simulink model "Quadrotor_14_step0_code_gen"  (Simulink 7.6)
settings: Solver=ode8  StartTime=0.0  StopTime=500  RelTol=1e-3
undefined symbols (not defined in the file): STARMAC, uav_utilities
libraries: aero_sim_lib x8, passive_control x1, simulink x1
settings Model: Creator=fluffy_bear  LastModifiedBy=jporter
settings OptimizationCC: BlockReduction=off  EnhancedBackFolding=on  OptimizeModelRefInitCode=on  LifeSpan=1
settings HardwareCC: ProdLargestAtomicInteger=Long  ProdLargestAtomicFloat=Float  ProdIntDivRoundTo=Floor  ProdEndianess=LittleEndian  ProdHWDeviceType=ARM Compatible->ARM 7
settings SFSimCC: SimParseCustomCode=off
settings RTWCC: SystemTargetFile=ert.tlc  GenCodeOnly=on  TemplateMakefile=ert_default_tmf  Description=Real-Time Workshop Embedded Coder  GenerateReport=on  ProcessScript=ert_make_rtw_hook  IncludeHyperlinkInReport=on  LaunchReport=on  CheckMdlBeforeBuild=Warning
settings CodeAppCC: IgnoreCustomStorageClasses=off  MATLABSourceComments=on
settings ERTTargetCC: MultiwordLength=2048  GenerateSampleERTMain=on  CombineSignalStateStructs=on  MultiInstanceERTCode=on  MultiInstanceErrorCode=Warning  ERTCustomFileTemplate=example_file_process.tlc  ConvertIfToSwitch=off

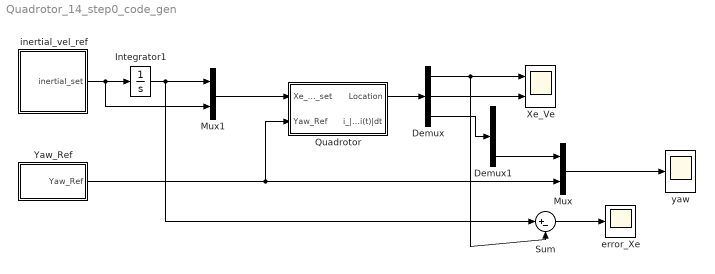
== system Quadrotor_14_step0_code_gen ==
  Demux : Demux  Outputs=[3,3,3]
  Demux1 : Demux  Outputs=3
  Integrator1 : Integrator
  Mux : Mux  Inputs=2
  Mux1 : Mux  Inputs=2
  Quadrotor : Subsystem  AncestorBlock=uav_utilities/STARMAC
  Sum : Sum  Inputs=|+-
  Xe_Ve : Scope  NumInputPorts=2
      settings: YMin=-100~-1.75  YMax=100~1.75  MaxDataPoints=100000  SampleInput=on  SampleTime=100/5000
  Yaw_Ref : Subsystem
  error_Xe : Scope
      settings: YMin=-9  SaveName=error_data  MaxDataPoints=20000  Decimation=10  SampleInput=on  SampleTime=100/5000
  inertial_vel_ref : Subsystem
  yaw : Scope
      settings: TimeRange=2  YMin=0.325  YMax=0.9  MaxDataPoints=100000  SampleInput=on  SampleTime=100/5000
  wires:
  inertial_vel_ref/1(inertial_set) -> Integrator1/1, Mux1/2
  Yaw_Ref/1(Yaw_Ref) -> Quadrotor/2(Yaw_Ref), Mux/2
  Sum/1 -> error_Xe/1
  Quadrotor/1(Location) -> Demux/1
  Demux/1 -> Sum/2, Xe_Ve/1
  Demux/2 -> Xe_Ve/2
  Mux/1 -> yaw/1
  Demux/3 -> Demux1/1
  Demux1/3 -> Mux/1
  Integrator1/1 -> Mux1/1, Sum/1
  Mux1/1 -> Quadrotor/1(Xe_Ve_set)

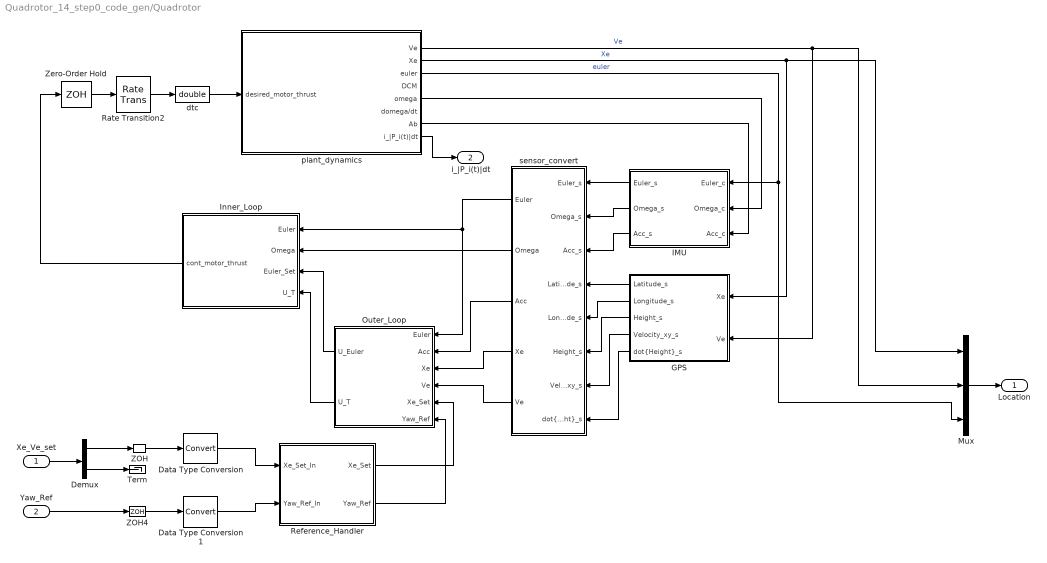
== system Quadrotor_14_step0_code_gen/Quadrotor ==
  Xe_Ve_set : Inport  PortDimensions=[6]
  Yaw_Ref : Inport  Port=2  PortDimensions=[1]
  Data Type Conversion : DataTypeConversion
  Data Type Conversion1 : DataTypeConversion
  Demux : Demux  Outputs=[3,3]
  GPS : Subsystem
  IMU : Subsystem
  Inner_Loop : Subsystem
  Mux : Mux  Inputs=[3 3 3]
  Outer_Loop : Subsystem
  Rate Transition2 : RateTransition
  Reference_Handler : Subsystem
  Term : Terminator
  ZOH : ZeroOrderHold  SampleTime=.01
  ZOH4 : ZeroOrderHold  SampleTime=.01
  Zero-Order Hold : ZeroOrderHold  SampleTime=.02
  dtc : DataTypeConversion  OutDataTypeStr=double
  plant_dynamics : Subsystem  AncestorBlock=aero_sim_lib/starmac_dynamics
  sensor_convert : Subsystem
  Location : Outport
  i_|P_i(t)|dt : Outport  Port=2
  wires:
  ZOH4/1 -> Data Type Conversion1/1
  Demux/2 -> Term/1
  Demux/1 -> ZOH/1
  Xe_Ve_set/1 -> Demux/1
  Mux/1 -> Location/1
  plant_dynamics/3(euler) -> Mux/3, IMU/1(Euler_c)  "euler"
  plant_dynamics/2(Xe) -> Mux/1, GPS/1(Xe)  "Xe"
  plant_dynamics/1(Ve) -> Mux/2, GPS/2(Ve)  "Ve"
  dtc/1 -> plant_dynamics/1(desired_motor_thrust)
  Zero-Order Hold/1 -> Rate Transition2/1
  Rate Transition2/1 -> dtc/1
  ZOH/1 -> Data Type Conversion/1
  plant_dynamics/5(omega) -> IMU/2(Omega_c)
  plant_dynamics/7(Ab) -> IMU/3(Acc_c)
  plant_dynamics/8(i_|P_i(t)|dt) -> i_|P_i(t)|dt/1
  Yaw_Ref/1 -> ZOH4/1
  IMU/1(Euler_s) -> sensor_convert/1(Euler_s)
  IMU/2(Omega_s) -> sensor_convert/2(Omega_s)
  IMU/3(Acc_s) -> sensor_convert/3(Acc_s)
  GPS/1(Latitude_s) -> sensor_convert/4(Latitude_s)
  GPS/2(Longitude_s) -> sensor_convert/5(Longitude_s)
  GPS/3(Height_s) -> sensor_convert/6(Height_s)
  GPS/4(Velocity_xy_s) -> sensor_convert/7(Velocity_xy_s)
  GPS/5("dot{Height}_s") -> sensor_convert/8("dot{Height}_s")
  Outer_Loop/1(U_Euler) -> Inner_Loop/3(Euler_Set)
  Outer_Loop/2(U_T) -> Inner_Loop/4(U_T)
  sensor_convert/1(Euler) -> Inner_Loop/1(Euler), Outer_Loop/1(Euler)
  sensor_convert/2(Omega) -> Inner_Loop/2(Omega)
  sensor_convert/3(Acc) -> Outer_Loop/2(Acc)
  sensor_convert/4(Xe) -> Outer_Loop/3(Xe)
  sensor_convert/5(Ve) -> Outer_Loop/4(Ve)
  Data Type Conversion/1 -> Reference_Handler/1(Xe_Set_In)
  Data Type Conversion1/1 -> Reference_Handler/2(Yaw_Ref_In)
  Reference_Handler/1(Xe_Set) -> Outer_Loop/5(Xe_Set)
  Reference_Handler/2(Yaw_Ref) -> Outer_Loop/6(Yaw_Ref)
  Inner_Loop/1(cont_motor_thrust) -> Zero-Order Hold/1

== system Quadrotor_14_step0_code_gen/Yaw_Ref ==
  Signal Generator : SignalGenerator  Frequency=2*.0625*0.25
  Yaw_Ref : Outport
  wires:
  Signal Generator/1 -> Yaw_Ref/1

== system Quadrotor_14_step0_code_gen/inertial_vel_ref ==
  Signal Generator : SignalGenerator  Amplitude=1.8*[1 -1 -.5]  Frequency=.1*.0625*ones(3,1)
  inertial_set : Outport
  wires:
  Signal Generator/1 -> inertial_set/1

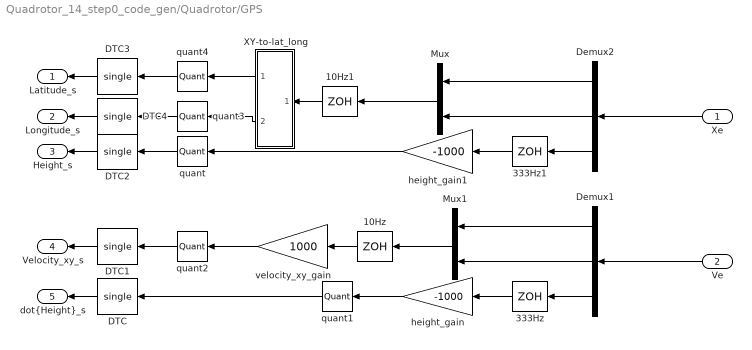
== system Quadrotor_14_step0_code_gen/Quadrotor/GPS ==
  Xe : Inport  OutDataTypeStr=double
  Ve : Inport  Port=2  OutDataTypeStr=double
  10Hz : ZeroOrderHold  SampleTime=.1
  10Hz1 : ZeroOrderHold  SampleTime=.1
  333Hz : ZeroOrderHold  SampleTime=1/333
  333Hz1 : ZeroOrderHold  SampleTime=1/333
  DTC{,1..4} (5 alike) : DataTypeConversion  OutDataTypeStr=single
  Demux1 : Demux  Outputs=[1,1,1]
  Demux2 : Demux  Outputs=[1,1,1]
  Mux : Mux  Inputs=2
  Mux1 : Mux  Inputs=2
  XY-to-lat_long : Subsystem  mask{lat_0=36.1658333, lon_0=-86.7844444}
  height_gain : Gain  Gain=-1000  RndMeth=Round  SaturateOnIntegerOverflow=on  OutDataTypeStr=Inherit: Same as input  LockScale=on
  height_gain1 : Gain  Gain=-1000  RndMeth=Round  SaturateOnIntegerOverflow=on  OutDataTypeStr=Inherit: Same as input  LockScale=on
  quant{,1,3..4} (4 alike) : Quantizer  QuantizationInterval=1
  quant2 : Quantizer  QuantizationInterval=ones(2,1)
  velocity_xy_gain : Gain  Gain=1000  RndMeth=Round  SaturateOnIntegerOverflow=on  OutDataTypeStr=Inherit: Same as input  LockScale=on
  Latitude_s : Outport
  Longitude_s : Outport  Port=2
  Height_s : Outport  Port=3
  Velocity_xy_s : Outport  Port=4
  "dot{Height}_s" : Outport  Port=5
  wires:
  Ve/1 -> Demux1/1
  Xe/1 -> Demux2/1
  Demux1/3 -> 333Hz/1
  Demux2/3 -> 333Hz1/1
  Demux2/1 -> Mux/1
  Demux2/2 -> Mux/2
  Demux1/1 -> Mux1/1
  Demux1/2 -> Mux1/2
  333Hz1/1 -> height_gain1/1
  333Hz/1 -> height_gain/1
  Mux1/1 -> 10Hz/1
  10Hz/1 -> velocity_xy_gain/1
  height_gain1/1 -> quant/1
  height_gain/1 -> quant1/1
  quant/1 -> DTC2/1
  quant1/1 -> DTC/1
  velocity_xy_gain/1 -> quant2/1
  quant2/1 -> DTC1/1
  10Hz1/1 -> XY-to-lat_long/1(XY)
  XY-to-lat_long/1(lat) -> quant4/1
  XY-to-lat_long/2(lon) -> quant3/1
  Mux/1 -> 10Hz1/1
  DTC/1 -> "dot{Height}_s"/1
  DTC1/1 -> Velocity_xy_s/1
  DTC2/1 -> Height_s/1
  DTC3/1 -> Latitude_s/1
  DTC4/1 -> Longitude_s/1
  quant3/1 -> DTC4/1
  quant4/1 -> DTC3/1

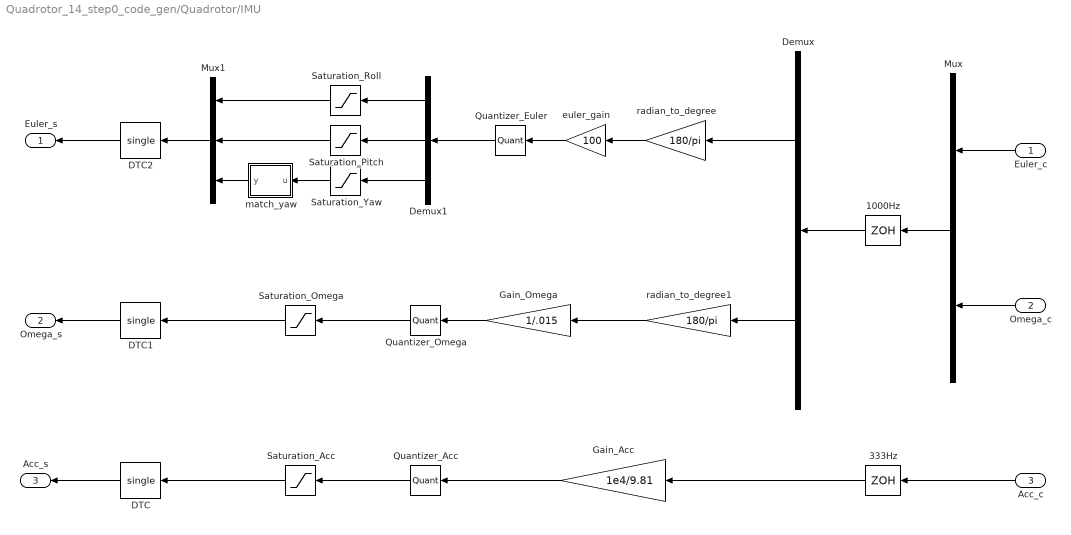
== system Quadrotor_14_step0_code_gen/Quadrotor/IMU ==
  Euler_c : Inport  OutDataTypeStr=double
  Omega_c : Inport  Port=2  OutDataTypeStr=double
  Acc_c : Inport  Port=3
  1000Hz : ZeroOrderHold  SampleTime=.001
  333Hz : ZeroOrderHold  SampleTime=1/333
  DTC : DataTypeConversion  OutDataTypeStr=single
  DTC1 : DataTypeConversion  OutDataTypeStr=single
  DTC2 : DataTypeConversion  OutDataTypeStr=single
  Demux : Demux  Outputs=[3,3]
  Demux1 : Demux  Outputs=[1,1,1]
  Gain_Acc : Gain  Gain=1e4/9.81
  Gain_Omega : Gain  Gain=1/.015
  Mux : Mux  Inputs=[3,3]
  Mux1 : Mux  Inputs=[1,1,1]
  Quantizer_Acc : Quantizer  QuantizationInterval=ones(3,1)
  Quantizer_Euler : Quantizer  QuantizationInterval=ones(3,1)
  Quantizer_Omega : Quantizer  QuantizationInterval=ones(3,1)
  Saturation_Acc : Saturate  UpperLimit=30000  LowerLimit=-30000  RndMeth=Round
      settings: LockScale=on
  Saturation_Omega : Saturate  UpperLimit=((2^15)-1) * ones(3,1)  LowerLimit=-(2^15) * ones(3,1)  OutDataTypeStr=double  RndMeth=Round
      settings: LockScale=on
  Saturation_Pitch : Saturate  UpperLimit=90*100  LowerLimit=-90*100  RndMeth=Round
      settings: LockScale=on
  Saturation_Roll : Saturate  UpperLimit=90*100  LowerLimit=-90*100  RndMeth=Round
      settings: LockScale=on
  Saturation_Yaw : Saturate  UpperLimit=180*100  LowerLimit=-180*100  RndMeth=Round
      settings: LockScale=on
  euler_gain : Gain  Gain=100
  match_yaw : Stateflow chart  TreatAsAtomicUnit=on
  radian_to_degree : Gain  Gain=180/pi
  radian_to_degree1 : Gain  Gain=180/pi
  Euler_s : Outport  LockScale=on
  Omega_s : Outport  Port=2  LockScale=on
  Acc_s : Outport  Port=3  LockScale=on
  wires:
  Mux/1 -> 1000Hz/1
  Euler_c/1 -> Mux/1
  1000Hz/1 -> Demux/1
  Gain_Acc/1 -> Quantizer_Acc/1
  Omega_c/1 -> Mux/2
  333Hz/1 -> Gain_Acc/1
  Saturation_Acc/1 -> DTC/1
  Saturation_Omega/1 -> DTC1/1
  Demux1/1 -> Saturation_Roll/1
  Saturation_Roll/1 -> Mux1/1
  Mux1/1 -> DTC2/1
  Demux1/2 -> Saturation_Pitch/1
  Saturation_Pitch/1 -> Mux1/2
  Demux1/3 -> Saturation_Yaw/1
  Saturation_Yaw/1 -> match_yaw/1(u)
  Gain_Omega/1 -> Quantizer_Omega/1
  Demux/1 -> radian_to_degree/1
  radian_to_degree/1 -> euler_gain/1
  Demux/2 -> radian_to_degree1/1
  euler_gain/1 -> Quantizer_Euler/1
  Quantizer_Euler/1 -> Demux1/1
  match_yaw/1(y) -> Mux1/3
  radian_to_degree1/1 -> Gain_Omega/1
  Quantizer_Omega/1 -> Saturation_Omega/1
  Acc_c/1 -> 333Hz/1
  Quantizer_Acc/1 -> Saturation_Acc/1
  DTC/1 -> Acc_s/1
  DTC1/1 -> Omega_s/1
  DTC2/1 -> Euler_s/1

== system Quadrotor_14_step0_code_gen/Quadrotor/Inner_Loop ==
  Euler : Inport  OutDataTypeStr=single
  Omega : Inport  Port=2  OutDataTypeStr=single
  Euler_Set : Inport  Port=3  OutDataTypeStr=single
  U_T : Inport  Port=4  OutDataTypeStr=single
  euler_controller : Subsystem  mask{K=1, K_e=7.5/.65, K_o=.5}
      mask prompts: K "Loop Gain [K]:"; K_e "Euler Gain [K_e]:"; K_o "Omega Gain [K_o]:"
  lead_motor : Subsystem  mask{tau_motor=.10, t_s=.01}
      mask init:
      | Hs=tf([tau_motor 1],[t_s/pi 1]);
      | Hz=ipesh_transform(Hs,t_s);
      | %a=1/tau_motor;
      | %b=pi/t_s;
      | %T=t_s;
      | %num1=b*(1-exp(-b*T))+a*(b*T-1+exp(-b*T));
      | %num2=-b*(1-exp(-b*T))+a*(1-exp(-b*T)-b*T*exp(-b*T));
      | %den1=a*b;
      | %den2=-a*b*exp(-b*T);
      | %num=[num1 num2];
      | %den=[den1 den2];
      | %Hz=tf(num,den,T);
      | %[y,t]=step(Hz);
      | %k_ss=(1/y(length(y)));
      | %num=k_ss*num;
      | %lead_a_1=single(-den(2)/den(1))
      | %lead_b_1=single(num(2)/den(1))
      | %lead_b_2=single(num(1)/den(1))
      | %Hz=k_ss*Hz
      | %bode(Hz);
  thrust_limit : Saturate  UpperLimit=10*ones(4,1)  LowerLimit=0*ones(4,1)  OutDataTypeStr=single
  u_T_u_torque_motor_thrust : Subsystem  mask{dx=.3048, K_torque=.47}
      mask prompts: dx "X distance of motor from CG [dx](meters):"; K_torque "Ktorque [K_torque]:"
      mask init:
      | M=[0 -dx 0 dx;
      |    dx 0 -dx 0;
      |    -K_torque K_torque -K_torque K_torque;
      |    1 1 1 1];
      | Mi=single(inv(M));
  cont_motor_thrust : Outport
  wires:
  Euler_Set/1 -> euler_controller/1(euler_set)
  U_T/1 -> u_T_u_torque_motor_thrust/2(u_T)
  euler_controller/1(u_torque) -> u_T_u_torque_motor_thrust/1(u_torque)
  thrust_limit/1 -> cont_motor_thrust/1
  u_T_u_torque_motor_thrust/1(cont_motor_thrust) -> lead_motor/1(thrust_in)
  lead_motor/1(thrust_out) -> thrust_limit/1
  Euler/1 -> euler_controller/2(euler)
  Omega/1 -> euler_controller/3(omega)

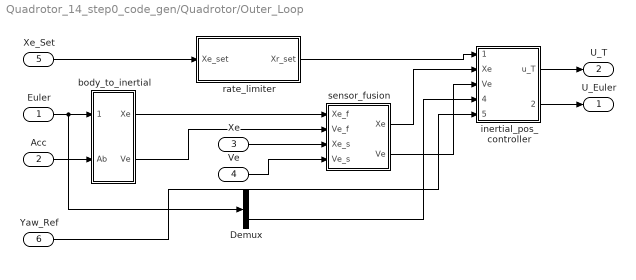
== system Quadrotor_14_step0_code_gen/Quadrotor/Outer_Loop ==
  Euler : Inport  OutDataTypeStr=single  PortDimensions=[3]
  Acc : Inport  Port=2  OutDataTypeStr=single  PortDimensions=[3]
  Xe : Inport  Port=3  OutDataTypeStr=single  PortDimensions=[3]
  Ve : Inport  Port=4  OutDataTypeStr=single  PortDimensions=[3]
  Xe_Set : Inport  Port=5  OutDataTypeStr=single  PortDimensions=[3]
  Yaw_Ref : Inport  Port=6  OutDataTypeStr=single  PortDimensions=[1]
  Demux : Demux  Outputs=3
  body_to_inertial : Subsystem
  inertial_pos_controller : Subsystem
  rate_limiter : Subsystem  mask{wn=2*pi, zeta=0.9, Vmax=2, T=0.01}
      mask prompts: wn "omega_n"; Vmax "Max velocity"; T "Sample time"
      mask init:
      | Hs=tf([wn^2],[1,2*zeta*wn,wn^2]);
      | Hz=ipesh_transform(Hs,T);
  sensor_fusion : Subsystem  mask{tau=.1, Ts=.01, Ts_gps=.1}
      mask prompts: tau "low-pass time constant (sec) [tau]"; Ts "Sample time [Ts]"; Ts_gps "GPS Sample Time [Ts_gps]"
  U_Euler : Outport  OutDataTypeStr=single  PortDimensions=[3]
  U_T : Outport  Port=2  OutDataTypeStr=single  PortDimensions=[1]
  wires:
  Xe_Set/1 -> rate_limiter/1(Xe_set)
  inertial_pos_controller/1(u_T) -> U_T/1
  inertial_pos_controller/2(u_euler) -> U_Euler/1
  Euler/1 -> body_to_inertial/1(euler), Demux/1
  Acc/1 -> body_to_inertial/2(Ab)
  sensor_fusion/1(Xe) -> inertial_pos_controller/2(Xe)
  sensor_fusion/2(Ve) -> inertial_pos_controller/3(Ve)
  body_to_inertial/1(Xe) -> sensor_fusion/1(Xe_f)
  body_to_inertial/2(Ve) -> sensor_fusion/2(Ve_f)
  Xe/1 -> sensor_fusion/3(Xe_s)
  Ve/1 -> sensor_fusion/4(Ve_s)
  rate_limiter/1(Xr_set) -> inertial_pos_controller/1(Xe_set)
  Demux/3 -> inertial_pos_controller/4(Yaw_actual)
  Yaw_Ref/1 -> inertial_pos_controller/5(Yaw_set)

== system Quadrotor_14_step0_code_gen/Quadrotor/Reference_Handler ==
  Xe_Set_In : Inport
  Yaw_Ref_In : Inport  Port=2
  Gain : Gain
  Gain1 : Gain
  Xe_Set : Outport
  Yaw_Ref : Outport  Port=2
  wires:
  Xe_Set_In/1 -> Gain/1
  Yaw_Ref_In/1 -> Gain1/1
  Gain1/1 -> Yaw_Ref/1
  Gain/1 -> Xe_Set/1

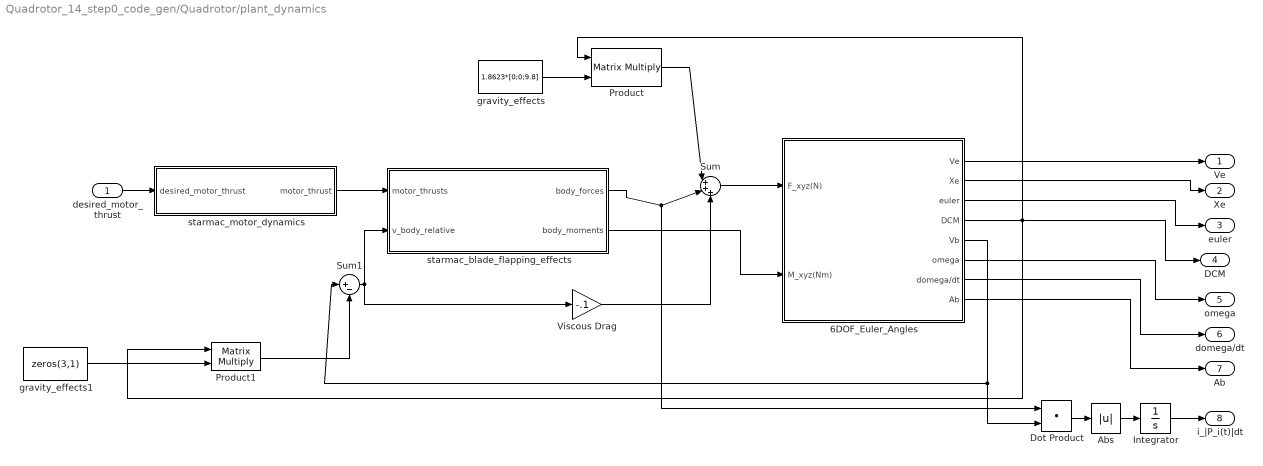
== system Quadrotor_14_step0_code_gen/Quadrotor/plant_dynamics ==
  desired_motor_thrust : Inport
  6DOF_Euler_Angles : Subsystem  AncestorBlock=aero_sim_lib/6DOF (Euler Angles)_CMU  mask{XYZe_0=[0.01;0.01;0], Vb_0=[0;0;0], euler_0=[0;0;0], omega_0=[0;0;0], M=1.8623, I=diag([0.02759 0.02771 0.04806])}
      mask prompts: XYZe_0 "Initial position in inertial axes [Xe,Ye,Ze]:"; Vb_0 "Initial velocity in body axes [U,v,w]:"; euler_0 "Initial Euler orientation [roll, pitch, yaw]=[phi,theta,psi]:"; omega_0 "Initial body rotation rates [p,q,r]=omega:"; M "Initial mass:"; I "Inertial:"
  Abs : Abs
  Dot Product : DotProduct  InputSameDT=on  OutDataTypeStr=Inherit: Inherit via internal rule
  Integrator : Integrator
  Product : Product  Multiplication=Matrix(*)  RndMeth=Zero
  Product1 : Product  Multiplication=Matrix(*)  RndMeth=Zero
  Sum : Sum  Inputs=|+++
  Sum1 : Sum  Inputs=|+-
  Viscous Drag : Gain  Gain=-.1
  gravity_effects : Constant  Value=1.8623*[0;0;9.8]
  gravity_effects1 : Constant  Value=zeros(3,1)  OutDataTypeStr=double
  starmac_blade_flapping_effects : Subsystem  AncestorBlock=aero_sim_lib/starmac_blade_flapping_effects
  starmac_motor_dynamics : Subsystem  AncestorBlock=aero_sim_lib/starmac_motor_dynamics  mask{tau_motor=.1, T_nom=1.8263*9.8/4, thrust_max=9.8, thrust_min=0, motor_lag_enable=on, motor_variance=.01*(.05*9.8/4)^2, Ts=1/76}
      mask prompts: tau_motor "tau_motor (seconds):"; T_nom "nominal thrust (N):"; thrust_max "maximum thrust (N):"; thrust_min "minimum thrust (N):"; motor_lag_enable "Motor Lag Enabled:"; motor_variance "Motor Variance [motor_variance]:"; Ts "Motor Update Rate (seconds):"
  Ve : Outport
  Xe : Outport  Port=2
  euler : Outport  Port=3
  DCM : Outport  Port=4
  omega : Outport  Port=5
  domega/dt : Outport  Port=6
  Ab : Outport  Port=7
  i_|P_i(t)|dt : Outport  Port=8
  wires:
  desired_motor_thrust/1 -> starmac_motor_dynamics/1(desired_motor_thrust)
  starmac_blade_flapping_effects/1(body_forces) -> Sum/2, Dot Product/1
  starmac_blade_flapping_effects/2(body_moments) -> 6DOF_Euler_Angles/2(M_xyz(Nm))
  Viscous Drag/1 -> Sum/3
  6DOF_Euler_Angles/5(Vb) -> Sum1/1, Dot Product/2
  Product1/1 -> Sum1/2
  Sum1/1 -> Viscous Drag/1, starmac_blade_flapping_effects/2(v_body_relative)
  gravity_effects/1 -> Product/2
  6DOF_Euler_Angles/4(DCM) -> Product1/1, Product/1, DCM/1
  Sum/1 -> 6DOF_Euler_Angles/1(F_xyz(N))
  Product/1 -> Sum/1
  starmac_motor_dynamics/1(motor_thrust) -> starmac_blade_flapping_effects/1(motor_thrusts)
  6DOF_Euler_Angles/1(Ve) -> Ve/1
  6DOF_Euler_Angles/2(Xe) -> Xe/1
  6DOF_Euler_Angles/3(euler) -> euler/1
  6DOF_Euler_Angles/6(omega) -> omega/1
  6DOF_Euler_Angles/7(domega/dt) -> domega/dt/1
  6DOF_Euler_Angles/8(Ab) -> Ab/1
  Integrator/1 -> i_|P_i(t)|dt/1
  Dot Product/1 -> Abs/1
  Abs/1 -> Integrator/1
  gravity_effects1/1 -> Product1/2

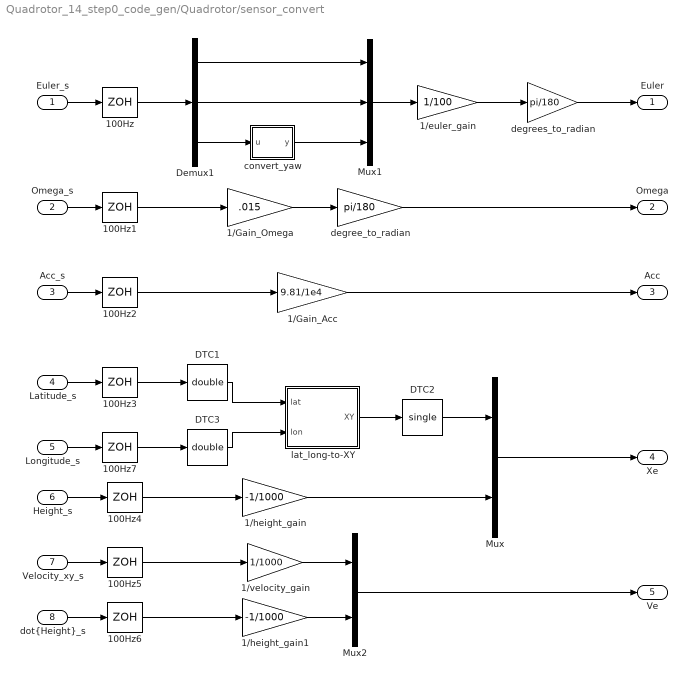
== system Quadrotor_14_step0_code_gen/Quadrotor/sensor_convert ==
  Euler_s : Inport
  Omega_s : Inport  Port=2
  Acc_s : Inport  Port=3
  Latitude_s : Inport  Port=4
  Longitude_s : Inport  Port=5
  Height_s : Inport  Port=6  OutDataTypeStr=single
  Velocity_xy_s : Inport  Port=7  OutDataTypeStr=single
  "dot{Height}_s" : Inport  Port=8  OutDataTypeStr=single
  1/Gain_Acc : Gain  Gain=9.81/1e4  OutDataTypeStr=single
  1/Gain_Omega : Gain  Gain=.015  OutDataTypeStr=single
  1/euler_gain : Gain  Gain=1/100
  1/height_gain : Gain  Gain=-1/1000
  1/height_gain1 : Gain  Gain=-1/1000
  1/velocity_gain : Gain  Gain=1/1000
  100Hz{,1..7} (8 alike) : ZeroOrderHold  SampleTime=.01
  DTC1 : DataTypeConversion  OutDataTypeStr=double
  DTC2 : DataTypeConversion  OutDataTypeStr=single
  DTC3 : DataTypeConversion  OutDataTypeStr=double
  Demux1 : Demux  Outputs=3
  Mux : Mux  Inputs=[2,1]
  Mux1 : Mux  Inputs=3
  Mux2 : Mux  Inputs=[2,1]
  convert_yaw : Stateflow chart  TreatAsAtomicUnit=on
  degree_to_radian : Gain  Gain=pi/180  OutDataTypeStr=single
  degrees_to_radian : Gain  Gain=pi/180  OutDataTypeStr=single
  lat_long-to-XY : Stateflow chart  TreatAsAtomicUnit=on
  Euler : Outport
  Omega : Outport  Port=2
  Acc : Outport  Port=3
  Xe : Outport  Port=4
  Ve : Outport  Port=5
  wires:
  Omega_s/1 -> 100Hz1/1
  1/Gain_Omega/1 -> degree_to_radian/1
  1/Gain_Acc/1 -> Acc/1
  Acc_s/1 -> 100Hz2/1
  100Hz2/1 -> 1/Gain_Acc/1
  100Hz1/1 -> 1/Gain_Omega/1
  degree_to_radian/1 -> Omega/1
  Euler_s/1 -> 100Hz/1
  100Hz/1 -> Demux1/1
  Mux1/1 -> 1/euler_gain/1
  degrees_to_radian/1 -> Euler/1
  1/euler_gain/1 -> degrees_to_radian/1
  Demux1/1 -> Mux1/1
  Demux1/2 -> Mux1/2
  convert_yaw/1(y) -> Mux1/3
  Demux1/3 -> convert_yaw/1(u)
  Velocity_xy_s/1 -> 100Hz5/1
  Height_s/1 -> 100Hz4/1
  100Hz4/1 -> 1/height_gain/1
  1/height_gain/1 -> Mux/2
  Latitude_s/1 -> 100Hz3/1
  Longitude_s/1 -> 100Hz7/1
  lat_long-to-XY/1(XY) -> DTC2/1
  Mux/1 -> Xe/1
  "dot{Height}_s"/1 -> 100Hz6/1
  100Hz6/1 -> 1/height_gain1/1
  100Hz5/1 -> 1/velocity_gain/1
  1/height_gain1/1 -> Mux2/2
  Mux2/1 -> Ve/1
  DTC2/1 -> Mux/1
  1/velocity_gain/1 -> Mux2/1
  DTC1/1 -> lat_long-to-XY/1(lat)
  DTC3/1 -> lat_long-to-XY/2(lon)
  100Hz3/1 -> DTC1/1
  100Hz7/1 -> DTC3/1

== system Quadrotor_14_step0_code_gen/Quadrotor/GPS/XY-to-lat_long ==
  XY : Inport
  XY-to-lat_long : Stateflow chart  TreatAsAtomicUnit=on
  lat : Outport
  lon : Outport  Port=2
  wires:
  XY-to-lat_long/1(lat) -> lat/1
  XY/1 -> XY-to-lat_long/1(XY)
  XY-to-lat_long/2(lon) -> lon/1

== system Quadrotor_14_step0_code_gen/Quadrotor/Inner_Loop/euler_controller ==
  euler_set : Inport
  euler : Inport  Port=2
  omega : Inport  Port=3
  K_euler : Gain  Gain=single(K_e)
  K_omega : Gain  Gain=single(K_o)  OutDataTypeStr=single
  SectorSearch : Subsystem  AncestorBlock=passive_control/SectorSearch
  Sum : Sum  Inputs=|+-  AccumDataTypeStr=single
  Sum1 : Sum  Inputs=|+-  AccumDataTypeStr=single
  euler_sector : Scope
      settings: TimeRange=80  YMin=-1  YMax=1  SaveName=euler_sector_data  MaxDataPoints=50000
  torque_limit : Saturate  UpperLimit=9.8*.3048*ones(3,1)  LowerLimit=-9.8*.3048*ones(3,1)  OutDataTypeStr=single
  u_torque : Outport
  wires:
  Sum/1 -> K_omega/1
  euler_set/1 -> Sum1/1  "euler_set"
  Sum1/1 -> K_euler/1
  euler/1 -> Sum1/2, SectorSearch/2(y)  "euler"
  K_euler/1 -> Sum/1, SectorSearch/1(x)  "u_omega"
  torque_limit/1 -> u_torque/1
  K_omega/1 -> torque_limit/1
  omega/1 -> Sum/2  "omega"
  SectorSearch/1(a) -> euler_sector/1

== system Quadrotor_14_step0_code_gen/Quadrotor/Inner_Loop/lead_motor ==
  thrust_in : Inport  OutDataTypeStr=single
  Demux : Demux
  Discrete Transfer Fcn{,1..3} (4 alike) : DiscreteTransferFcn  Numerator=Hz.num{1}  Denominator=Hz.den{1}  SampleTime=-1
  Mux : Mux
  thrust_out : Outport  OutDataTypeStr=single
  wires:
  thrust_in/1 -> Demux/1  "x"
  Demux/1 -> Discrete Transfer Fcn/1
  Demux/2 -> Discrete Transfer Fcn1/1
  Demux/3 -> Discrete Transfer Fcn2/1
  Mux/1 -> thrust_out/1
  Discrete Transfer Fcn/1 -> Mux/1
  Discrete Transfer Fcn1/1 -> Mux/2
  Discrete Transfer Fcn2/1 -> Mux/3
  Demux/4 -> Discrete Transfer Fcn3/1
  Discrete Transfer Fcn3/1 -> Mux/4

== system Quadrotor_14_step0_code_gen/Quadrotor/Inner_Loop/u_T_u_torque_motor_thrust ==
  u_torque : Inport
  u_T : Inport  Port=2
  Mi : Gain  Gain=Mi  Multiplication=Matrix(K*u)  ParamDataTypeStr=single  OutDataTypeStr=single
  u_torque_u_T_mux : Stateflow chart  TreatAsAtomicUnit=on
  cont_motor_thrust : Outport
  wires:
  u_torque/1 -> u_torque_u_T_mux/1(u_torque)
  u_T/1 -> u_torque_u_T_mux/2(u_T)
  Mi/1 -> cont_motor_thrust/1
  u_torque_u_T_mux/1(u_torque_u_T) -> Mi/1

== system Quadrotor_14_step0_code_gen/Quadrotor/Outer_Loop/body_to_inertial ==
  euler : Inport
  Ab : Inport  Port=2
  Ab_to_Ae : Stateflow chart  TreatAsAtomicUnit=on
  inertial_vel_and pos_est : Subsystem  mask{Ts=.01}
      mask prompts: Ts "Sample Time [Ts] (seconds):"
  Xe : Outport
  Ve : Outport  Port=2
  wires:
  euler/1 -> Ab_to_Ae/1(euler)
  Ab/1 -> Ab_to_Ae/2(Ab)
  Ab_to_Ae/1(Ae) -> inertial_vel_and pos_est/1(Ab)
  inertial_vel_and pos_est/1(Vb) -> Ve/1
  inertial_vel_and pos_est/2(Xb) -> Xe/1

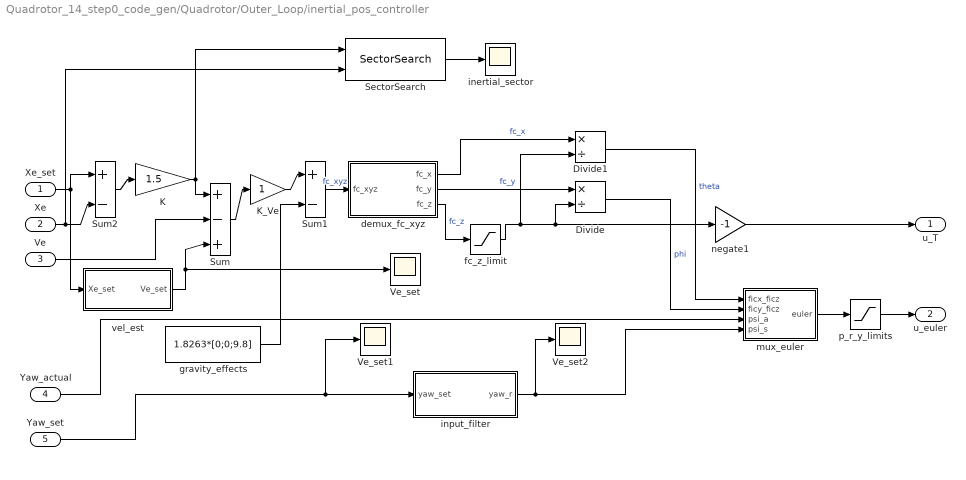
== system Quadrotor_14_step0_code_gen/Quadrotor/Outer_Loop/inertial_pos_controller ==
  Xe_set : Inport
  Xe : Inport  Port=2
  Ve : Inport  Port=3
  Yaw_actual : Inport  Port=4
  Yaw_set : Inport  Port=5
  Divide : Product  Inputs=*/  OutDataTypeStr=single
  Divide1 : Product  Inputs=*/  OutDataTypeStr=single
  K : Gain  Gain=1.5  OutDataTypeStr=single
  K_Ve : Gain  ParamDataTypeStr=single  OutDataTypeStr=single
  SectorSearch : passive_control/SectorSearch  SystemSampleTime=-1
  Sum : Sum  Inputs=|+-+  AccumDataTypeStr=single  OutDataTypeStr=single
  Sum1 : Sum  Inputs=|+-  AccumDataTypeStr=single  OutDataTypeStr=single
  Sum2 : Sum  Inputs=|+-  AccumDataTypeStr=single  OutDataTypeStr=single
  Ve_set : Scope
      settings: TimeRange=60  YMin=-1.75  YMax=2.25  SaveName=ScopeData2  Decimation=10
  Ve_set1 : Scope
      settings: TimeRange=60  SaveName=ScopeData10  Decimation=10
  Ve_set2 : Scope
      settings: TimeRange=60  SaveName=ScopeData11  Decimation=10
  demux_fc_xyz : Stateflow chart  TreatAsAtomicUnit=on
  fc_z_limit : Saturate  UpperLimit=-(1/8)*9.81  LowerLimit=-4*9.81  OutDataTypeStr=single
  gravity_effects : Constant  Value=1.8263*[0;0;9.8]  OutDataTypeStr=single
  inertial_sector : Scope
      settings: TimeRange=80  YMin=-1  YMax=1  SaveName=inertial_sector_data  MaxDataPoints=50000
  input_filter : Subsystem  mask{wn=1, zeta=0.9, T=0.01}
      mask prompts: wn "omega_n"; T "Sample time"
      mask init:
      | Hs=tf([wn^2],[1,2*zeta*wn,wn^2]);
      | Hz=ipesh_transform(Hs,T);
  mux_euler : Stateflow chart  TreatAsAtomicUnit=on
  negate1 : Gain  Gain=-1  OutDataTypeStr=single
  p_r_y_limits : Saturate  UpperLimit=[pi/4,pi/4,inf]  LowerLimit=-[pi/4,pi/4,inf]  OutDataTypeStr=single
  vel_est : Subsystem  mask{tau_f=.01/pi, T=.01}
      mask prompts: T "sample rate"
      mask init:
      | %b=1/tau_f;
      | %num1=(1-exp(-b*T));
      | %num2=-num1;
      | %den1=1;
      | %den2=-exp(-b*T);
      | %num=(1/T)*[num1 num2];
      | %den=[den1 den2];
      | %vel_est_a_1=single(-den(2)/den(1))
      | %vel_est_b_1=single(num(2)/den(1))
      | %vel_est_b_2=single(num(1)/den(1))
      | Hs=tf([1 0],[T/pi 1]);
      | Hz=ipesh_transform(Hs,T);
      | %Hz=tf(num,den,T);
      | %bode(Hz);
      | %hold on;
      | %bode(tf([1 0],[tau_f 1]));
  u_T : Outport
  u_euler : Outport  Port=2
  wires:
  fc_z_limit/1 -> Divide1/2, Divide/2, negate1/1
  Xe_set/1 -> Sum2/1, vel_est/1(Xe_set)
  negate1/1 -> u_T/1
  p_r_y_limits/1 -> u_euler/1
  demux_fc_xyz/1(fc_x) -> Divide1/1  "fc_x"
  demux_fc_xyz/3(fc_z) -> fc_z_limit/1  "fc_z"
  mux_euler/1(euler) -> p_r_y_limits/1
  Sum1/1 -> demux_fc_xyz/1(fc_xyz)  "fc_xyz"
  gravity_effects/1 -> Sum1/2
  Sum/1 -> K_Ve/1
  Xe/1 -> Sum2/2, SectorSearch/2
  Sum2/1 -> K/1
  K/1 -> Sum/1, SectorSearch/1
  demux_fc_xyz/2(fc_y) -> Divide/1  "fc_y"
  K_Ve/1 -> Sum1/1
  Ve/1 -> Sum/2
  vel_est/1(Ve_set) -> Sum/3, Ve_set/1
  Divide1/1 -> mux_euler/1(ficx_ficz)  "theta"
  Divide/1 -> mux_euler/2(ficy_ficz)  "phi"
  input_filter/1(yaw_r) -> Ve_set2/1, mux_euler/4(psi_s)
  Yaw_set/1 -> input_filter/1(yaw_set), Ve_set1/1
  Yaw_actual/1 -> mux_euler/3(psi_a)
  SectorSearch/1 -> inertial_sector/1

== system Quadrotor_14_step0_code_gen/Quadrotor/Outer_Loop/rate_limiter ==
  Xe_set : Inport
  Constant : Constant  Value=T  OutDataTypeStr=single
  Constant1 : Constant  Value=Vmax  OutDataTypeStr=single
  Demux : Demux  Outputs=3
  Discrete Transfer Fcn : DiscreteTransferFcn  Numerator=Hz.num{1}  Denominator=Hz.den{1}  SampleTime=-1
  Discrete Transfer Fcn1 : DiscreteTransferFcn  Numerator=Hz.num{1}  Denominator=Hz.den{1}  SampleTime=-1
  Discrete Transfer Fcn2 : DiscreteTransferFcn  Numerator=Hz.num{1}  Denominator=Hz.den{1}  SampleTime=-1
  Embedded MATLAB Function : Stateflow chart  TreatAsAtomicUnit=on
  Mux : Mux  Inputs=3
  Unit Delay : UnitDelay  SampleTime=-1
  Xr_set : Outport
  wires:
  Xe_set/1 -> Demux/1
  Mux/1 -> Embedded MATLAB Function/1(Xd)
  Embedded MATLAB Function/1(Xr) -> Xr_set/1, Unit Delay/1
  Unit Delay/1 -> Embedded MATLAB Function/2(Xd_prev)
  Constant/1 -> Embedded MATLAB Function/3(Tsamp)
  Constant1/1 -> Embedded MATLAB Function/4(Vmax)
  Demux/1 -> Discrete Transfer Fcn/1
  Discrete Transfer Fcn/1 -> Mux/1
  Demux/2 -> Discrete Transfer Fcn1/1
  Discrete Transfer Fcn1/1 -> Mux/2
  Demux/3 -> Discrete Transfer Fcn2/1
  Discrete Transfer Fcn2/1 -> Mux/3

== system Quadrotor_14_step0_code_gen/Quadrotor/Outer_Loop/sensor_fusion ==
  Xe_f : Inport
  Ve_f : Inport  Port=2
  Xe_s : Inport  Port=3
  Ve_s : Inport  Port=4
  anti-aliasing : Subsystem  mask{tau=tau, Ts=Ts}
      mask prompts: tau "tau (sec)"; Ts "Ts (sec)"
      mask init:
      | Hs = tf(1,[tau,1]);
      | Hz = ipesh_transform(Hs,Ts);
  sensor_fusion : Stateflow chart  TreatAsAtomicUnit=on
  Xe : Outport
  Ve : Outport  Port=2
  wires:
  Xe_f/1 -> sensor_fusion/2(Xe_f)
  Ve_f/1 -> sensor_fusion/4(Ve_f)
  sensor_fusion/1(Xe) -> anti-aliasing/1(u)
  anti-aliasing/1(y) -> Xe/1
  Xe_s/1 -> sensor_fusion/1(Xe_s)
  sensor_fusion/2(Ve) -> Ve/1
  Ve_s/1 -> sensor_fusion/3(Ve_s)

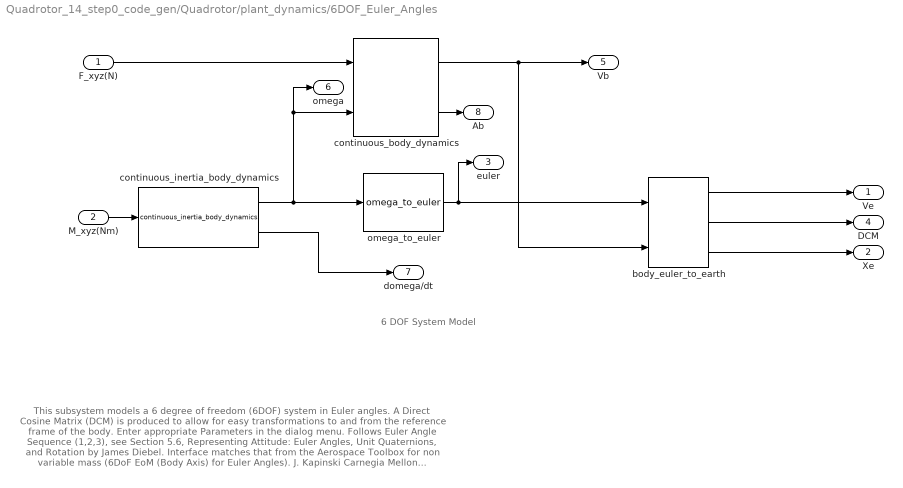
== system Quadrotor_14_step0_code_gen/Quadrotor/plant_dynamics/6DOF_Euler_Angles ==
  note: This subsystem models a 6 degree of freedom (6DOF) system in Euler angles.
      | A Direct Cosine Matrix (DCM) is produced to allow for easy transformations to
      | and from the reference frame of the body.  Enter appropriate Parameters in the dialog menu.
      | Follows Euler Angle Sequence (1,2,3), see Section 5.6, Representing Attitude: Euler Angles, Unit
      | Quaternions, and Rotation by James Diebel.  Interface matches that from the Aerospace Toolbox
      | for non variable mass (6DoF EoM (Body Axis) for Euler Angles).
      |
      | J. Kapinski
      | Carnegia Mellon University
      | 7/2007
      | Revised:
      | Nicholas Kottenstette, ISIS, 8/2008
  note: 6 DOF System Model
  F_xyz(N) : Inport
  M_xyz(Nm) : Inport  Port=2  PortDimensions=3
  body_euler_to_earth : aero_sim_lib/body_euler_to_earth  SystemSampleTime=-1  XYZe_0=XYZe_0
  continuous_body_dynamics : aero_sim_lib/continuous_body_dynamics  SystemSampleTime=-1  M=M  Vb_0=Vb_0
  continuous_inertia_body_dynamics : aero_sim_lib/continuous_inertia_body_dynamics  SystemSampleTime=-1  I=I  omega_0=omega_0
  omega_to_euler : aero_sim_lib/omega_to_euler  SystemSampleTime=-1  euler_0=euler_0
  Ve : Outport
  Xe : Outport  Port=2
  euler : Outport  Port=3
  DCM : Outport  Port=4
  Vb : Outport  Port=5
  omega : Outport  Port=6
  domega/dt : Outport  Port=7
  Ab : Outport  Port=8
  wires:
  body_euler_to_earth/3 -> Xe/1
  body_euler_to_earth/2 -> DCM/1
  body_euler_to_earth/1 -> Ve/1
  omega_to_euler/1 -> body_euler_to_earth/1, euler/1
  continuous_inertia_body_dynamics/2 -> domega/dt/1
  continuous_body_dynamics/2 -> Ab/1
  continuous_body_dynamics/1 -> body_euler_to_earth/2, Vb/1
  continuous_inertia_body_dynamics/1 -> omega_to_euler/1, continuous_body_dynamics/2, omega/1
  F_xyz(N)/1 -> continuous_body_dynamics/1
  M_xyz(Nm)/1 -> continuous_inertia_body_dynamics/1

== system Quadrotor_14_step0_code_gen/Quadrotor/plant_dynamics/starmac_blade_flapping_effects ==
  motor_thrusts : Inport
  v_body_relative : Inport  Port=2
  Pick First 2 Elements : Constant  Value=[1 0 0; 0 1 0; 0 0 0]
  Product : Product  RndMeth=Zero
  Product2 : Product  Multiplication=Matrix(*)  RndMeth=Zero
  Product4 : Product  RndMeth=Zero
  Sum : Sum  Inputs=|++
  Sum of Elements : Sum  Inputs=+
  starmac_body_moments : Subsystem  AncestorBlock=aero_sim_lib/starmac_body_moments  mask{dx=.3048, dz=.07, K_torque=.47}
  starmac_flapping_dynamics : Subsystem  AncestorBlock=aero_sim_lib/starmac_flapping_dynamics  mask{K_a1s=.009, K_beta=.23}
  starmac_vertical_effect_dynamics : Subsystem  AncestorBlock=aero_sim_lib/starmac_vertical_effect_dynamics  mask{tau_motor=0.1, R=0.127, Alpha=(pi/180)*[-85:5:85], Vinf=[0:0.5:6], Thrust=9.8*[0.3:0.02:0.8]}
      mask prompts: tau_motor "motor time constant (s)"; R "radius of propeller (m)"; Alpha "Alpha (radians)"; Vinf "Vinf (radians)"; Thrust "Propeller Thrust (N)"
      mask init:
      | rho = 1.2;
      | A = pi*R^2;
      | Vh = sqrt(Thrust/(2*rho*A));
      | for i = 1:length(Vh)
      |     for j = 1:length(Vinf)
      |         for k = 1:length(Alpha)
      |             Vi(k,j,i) = find_vi(Vh(i),Vinf(j),Alpha(k));
      |             ToverTh(k,j,i) = min(10,max(0.1,Vh(i)/(Vi(k,j,i)+Vinf(j)*sin(Alpha(k)))));
      |         end
      |     end
      | end
  body_forces : Outport
  body_moments : Outport  Port=2
  wires:
  starmac_flapping_dynamics/2(rotor_blade_moments) -> Sum/2
  Sum/1 -> body_moments/1
  starmac_body_moments/1(Body Moments) -> Sum/1
  starmac_flapping_dynamics/1(thrust_vector) -> Product4/2, starmac_body_moments/2(Thrust Vector)
  Product4/1 -> body_forces/1
  Sum of Elements/1 -> Product4/1
  Product2/1 -> starmac_flapping_dynamics/1(Vb2_hat)
  v_body_relative/1 -> Product2/2, starmac_vertical_effect_dynamics/2(v_body_relative)
  Pick First 2 Elements/1 -> Product2/1
  motor_thrusts/1 -> Product/1, starmac_vertical_effect_dynamics/1(motor_thrusts)
  starmac_vertical_effect_dynamics/1(thrust_multiplier) -> Product/2
  Product/1 -> Sum of Elements/1, starmac_body_moments/1(Thrust Magnitudes)

== system Quadrotor_14_step0_code_gen/Quadrotor/plant_dynamics/starmac_motor_dynamics ==
  desired_motor_thrust : Inport
  Band-Limited White Noise : simulink/Sources/Band-Limited White Noise  SystemSampleTime=-1  Cov=Ts*motor_variance*ones(4,1)  Ts=Ts  seed=22341+[0 1 2 3]'
  Constant : Constant  Value=motor_lag_enable
  Saturation : Saturate  UpperLimit=thrust_max*ones(4,1)  LowerLimit=thrust_min*ones(4,1)
  State-Space : StateSpace  A=-(1/tau_motor)*eye(4)  B=(1/tau_motor)*eye(4)  C=eye(4)  D=zeros(4,4)  X0=T_nom*ones(4,1)
  Sum : Sum  Inputs=|++
  Switch : Switch  Criteria=u2 > Threshold
  motor_thrust : Outport
  wires:
  desired_motor_thrust/1 -> State-Space/1, Switch/3
  Sum/1 -> motor_thrust/1
  Saturation/1 -> Sum/1
  Band-Limited White Noise/1 -> Sum/2
  State-Space/1 -> Switch/1
  Switch/1 -> Saturation/1
  Constant/1 -> Switch/2

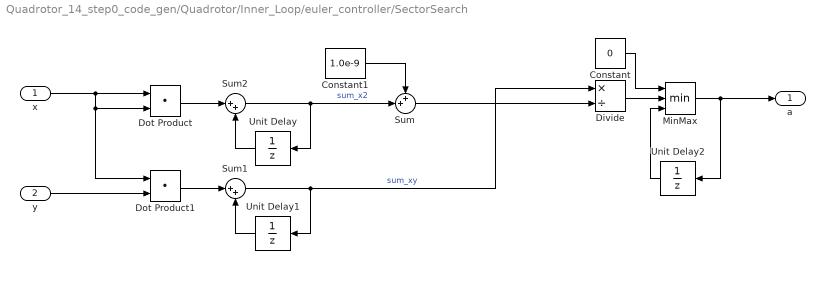
== system Quadrotor_14_step0_code_gen/Quadrotor/Inner_Loop/euler_controller/SectorSearch ==
  x : Inport
  y : Inport  Port=2
  Constant : Constant  Value=0
  Constant1 : Constant  Value=1.0e-9
  Divide : Product  Inputs=*/
  Dot Product : DotProduct  InputSameDT=on  OutDataTypeStr=Inherit: Inherit via internal rule
  Dot Product1 : DotProduct  InputSameDT=on  OutDataTypeStr=Inherit: Inherit via internal rule
  MinMax : MinMax  Inputs=3
  Sum : Sum  Inputs=++|
  Sum1 : Sum  Inputs=|++
  Sum2 : Sum  Inputs=|++
  Unit Delay : UnitDelay  SampleTime=-1
  Unit Delay1 : UnitDelay  SampleTime=-1
  Unit Delay2 : UnitDelay  SampleTime=-1
  a : Outport
  wires:
  Constant1/1 -> Sum/1
  Sum/1 -> Divide/2
  Unit Delay2/1 -> MinMax/3
  Divide/1 -> MinMax/2
  Constant/1 -> MinMax/1
  MinMax/1 -> a/1, Unit Delay2/1
  y/1 -> Dot Product1/2
  x/1 -> Dot Product1/1, Dot Product/2, Dot Product/1
  Dot Product1/1 -> Sum1/1
  Unit Delay1/1 -> Sum1/2
  Sum1/1 -> Divide/1, Unit Delay1/1  "sum_xy"
  Dot Product/1 -> Sum2/1
  Unit Delay/1 -> Sum2/2
  Sum2/1 -> Sum/2, Unit Delay/1  "sum_x2"

== system Quadrotor_14_step0_code_gen/Quadrotor/Outer_Loop/body_to_inertial/inertial_vel_and pos_est ==
  Ab : Inport
  DT_integrator : Subsystem
  DT_integrator1 : Subsystem
  Vb : Outport
  Xb : Outport  Port=2
  wires:
  DT_integrator1/1(Xb) -> Xb/1
  Ab/1 -> DT_integrator/1(Ab)
  DT_integrator/1(Vb) -> Vb/1, DT_integrator1/1(Vb)

== system Quadrotor_14_step0_code_gen/Quadrotor/Outer_Loop/inertial_pos_controller/input_filter ==
  yaw_set : Inport
  Discrete Transfer Fcn : DiscreteTransferFcn  Numerator=Hz.num{1}  Denominator=Hz.den{1}  SampleTime=-1
  yaw_r : Outport
  wires:
  yaw_set/1 -> Discrete Transfer Fcn/1
  Discrete Transfer Fcn/1 -> yaw_r/1

== system Quadrotor_14_step0_code_gen/Quadrotor/Outer_Loop/inertial_pos_controller/vel_est ==
  Xe_set : Inport
  Demux : Demux  Outputs=3
  Discrete Transfer Fcn : DiscreteTransferFcn  Numerator=Hz.num{1}  Denominator=Hz.den{1}  SampleTime=-1
  Discrete Transfer Fcn1 : DiscreteTransferFcn  Numerator=Hz.num{1}  Denominator=Hz.den{1}  SampleTime=-1
  Discrete Transfer Fcn2 : DiscreteTransferFcn  Numerator=Hz.num{1}  Denominator=Hz.den{1}  SampleTime=-1
  Mux : Mux  Inputs=3
  Ve_set : Outport
  wires:
  Xe_set/1 -> Demux/1  "x"
  Demux/1 -> Discrete Transfer Fcn/1
  Demux/2 -> Discrete Transfer Fcn1/1
  Demux/3 -> Discrete Transfer Fcn2/1
  Mux/1 -> Ve_set/1
  Discrete Transfer Fcn/1 -> Mux/1
  Discrete Transfer Fcn1/1 -> Mux/2
  Discrete Transfer Fcn2/1 -> Mux/3

== system Quadrotor_14_step0_code_gen/Quadrotor/Outer_Loop/sensor_fusion/anti-aliasing ==
  u : Inport
  Demux : Demux  Outputs=3
  Mux : Mux  Inputs=3
  smoothing-filter : DiscreteTransferFcn  Numerator=Hz.num{1}  Denominator=Hz.den{1}  SampleTime=-1
  smoothing-filter1 : DiscreteTransferFcn  Numerator=Hz.num{1}  Denominator=Hz.den{1}  SampleTime=-1
  y : Outport
  wires:
  Demux/3 -> Mux/3
  Demux/2 -> smoothing-filter1/1
  smoothing-filter1/1 -> Mux/2
  smoothing-filter/1 -> Mux/1
  Demux/1 -> smoothing-filter/1
  Mux/1 -> y/1
  u/1 -> Demux/1

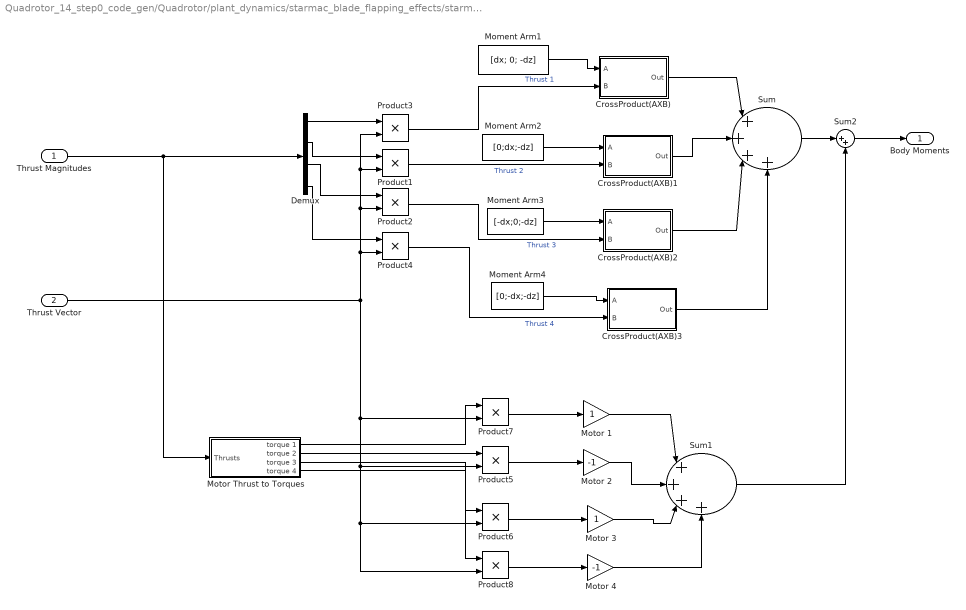
== system Quadrotor_14_step0_code_gen/Quadrotor/plant_dynamics/starmac_blade_flapping_effects/starmac_body_moments ==
  Thrust Magnitudes : Inport
  Thrust Vector : Inport  Port=2
  CrossProduct(AXB) : Subsystem
  CrossProduct(AXB)1 : Subsystem
  CrossProduct(AXB)2 : Subsystem
  CrossProduct(AXB)3 : Subsystem
  Demux : Demux
  Moment Arm1 : Constant  Value=[dx; 0; -dz]
  Moment Arm2 : Constant  Value=[0;dx;-dz]
  Moment Arm3 : Constant  Value=[-dx;0;-dz]
  Moment Arm4 : Constant  Value=[0;-dx;-dz]
  Motor 1 : Gain
  Motor 2 : Gain  Gain=-1
  Motor 3 : Gain
  Motor 4 : Gain  Gain=-1
  Motor Thrust to Torques : Subsystem
  Product{1..8} (8 alike) : Product  RndMeth=Zero
  Sum : Sum  Inputs=|++++
  Sum1 : Sum  Inputs=|++++
  Sum2 : Sum  Inputs=|++
  Body Moments : Outport
  wires:
  CrossProduct(AXB)1/1(Out) -> Sum/2
  Motor Thrust to Torques/4(torque 4) -> Product8/1
  Motor Thrust to Torques/3(torque 3) -> Product6/1
  Motor Thrust to Torques/2(torque 2) -> Product5/1
  Motor Thrust to Torques/1(torque 1) -> Product7/1
  Product8/1 -> Motor 4/1
  Product6/1 -> Motor 3/1
  Product5/1 -> Motor 2/1
  Product7/1 -> Motor 1/1
  Sum2/1 -> Body Moments/1
  Sum1/1 -> Sum2/2
  Sum/1 -> Sum2/1
  Motor 4/1 -> Sum1/4
  Motor 3/1 -> Sum1/3
  Motor 2/1 -> Sum1/2
  Motor 1/1 -> Sum1/1
  CrossProduct(AXB)3/1(Out) -> Sum/4
  CrossProduct(AXB)2/1(Out) -> Sum/3
  CrossProduct(AXB)/1(Out) -> Sum/1
  Product4/1 -> CrossProduct(AXB)3/2(B)  "Thrust 4"
  Moment Arm4/1 -> CrossProduct(AXB)3/1(A)
  Product2/1 -> CrossProduct(AXB)2/2(B)  "Thrust 3"
  Moment Arm3/1 -> CrossProduct(AXB)2/1(A)
  Product1/1 -> CrossProduct(AXB)1/2(B)  "Thrust 2"
  Moment Arm2/1 -> CrossProduct(AXB)1/1(A)
  Product3/1 -> CrossProduct(AXB)/2(B)  "Thrust 1"
  Moment Arm1/1 -> CrossProduct(AXB)/1(A)
  Thrust Vector/1 -> Product8/2, Product6/2, Product5/2, Product7/2, Product4/2, Product2/2, Product1/2, Product3/2
  Demux/4 -> Product4/1
  Demux/3 -> Product2/1
  Demux/2 -> Product1/1
  Demux/1 -> Product3/1
  Thrust Magnitudes/1 -> Motor Thrust to Torques/1(Thrusts), Demux/1

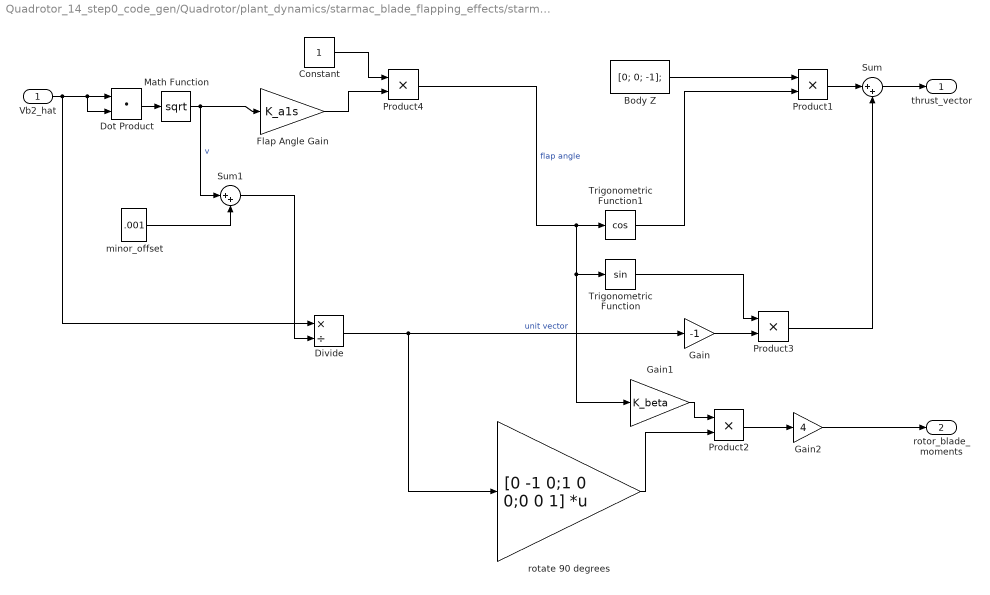
== system Quadrotor_14_step0_code_gen/Quadrotor/plant_dynamics/starmac_blade_flapping_effects/starmac_flapping_dynamics ==
  Vb2_hat : Inport
  "Body Z " : Constant  Value=[0; 0; -1];
  Constant : Constant
  Divide : Product  Inputs=*/
  Dot Product : DotProduct  InputSameDT=on  OutDataTypeStr=Inherit: Inherit via internal rule
  Flap Angle Gain : Gain  Gain=K_a1s
  Gain : Gain  Gain=-1
  Gain1 : Gain  Gain=K_beta
  Gain2 : Gain  Gain=4
  Math Function : Math  Operator=sqrt  SaturateOnIntegerOverflow=on
  Product{1..4} (4 alike) : Product  RndMeth=Zero
  Sum : Sum  Inputs=|++
  Sum1 : Sum  Inputs=|++
  Trigonometric Function : Trigonometry
  Trigonometric Function1 : Trigonometry  Operator=cos
  minor_offset : Constant  Value=.001
  rotate 90 degrees : Gain  Gain=[0 -1 0;1 0 0;0 0 1]  Multiplication=Matrix(K*u)
  thrust_vector : Outport
  rotor_blade_moments : Outport  Port=2
  wires:
  minor_offset/1 -> Sum1/2
  Sum1/1 -> Divide/2
  Divide/1 -> rotate 90 degrees/1, Gain/1  "unit vector"
  Product4/1 -> Trigonometric Function1/1, Trigonometric Function/1, Gain1/1  "flap angle"
  Vb2_hat/1 -> Divide/1, Dot Product/1, Dot Product/2
  Dot Product/1 -> Math Function/1
  Math Function/1 -> Sum1/1, Flap Angle Gain/1  "v"
  Trigonometric Function1/1 -> Product1/2
  Trigonometric Function/1 -> Product3/1
  Product3/1 -> Sum/2
  Gain/1 -> Product3/2
  Product1/1 -> Sum/1
  "Body Z "/1 -> Product1/1
  Sum/1 -> thrust_vector/1
  Gain2/1 -> rotor_blade_moments/1
  Product2/1 -> Gain2/1
  rotate 90 degrees/1 -> Product2/2
  Gain1/1 -> Product2/1
  Flap Angle Gain/1 -> Product4/2
  Constant/1 -> Product4/1

== system Quadrotor_14_step0_code_gen/Quadrotor/plant_dynamics/starmac_blade_flapping_effects/starmac_vertical_effect_dynamics ==
  motor_thrusts : Inport
  v_body_relative : Inport  Port=2
  Demux : Demux
  Mux : Mux
  starmac_motor_vertical_effect_dynamics{,1..3} (4 alike) : aero_sim_lib/starmac_motor_vertical_effect_dynamics  SystemSampleTime=-1  tau_motor=tau_motor  R=R  Alpha=Alpha  Vinf=Vinf  Vh=Vh  ToverTh=ToverTh
  thrust_multiplier : Outport
  wires:
  motor_thrusts/1 -> Demux/1
  Mux/1 -> thrust_multiplier/1
  Demux/1 -> starmac_motor_vertical_effect_dynamics/1
  Demux/2 -> starmac_motor_vertical_effect_dynamics1/1
  Demux/3 -> starmac_motor_vertical_effect_dynamics2/1
  Demux/4 -> starmac_motor_vertical_effect_dynamics3/1
  starmac_motor_vertical_effect_dynamics/1 -> Mux/1
  starmac_motor_vertical_effect_dynamics1/1 -> Mux/2
  starmac_motor_vertical_effect_dynamics2/1 -> Mux/3
  starmac_motor_vertical_effect_dynamics3/1 -> Mux/4
  v_body_relative/1 -> starmac_motor_vertical_effect_dynamics2/2, starmac_motor_vertical_effect_dynamics3/2, starmac_motor_vertical_effect_dynamics1/2, starmac_motor_vertical_effect_dynamics/2

== system Quadrotor_14_step0_code_gen/Quadrotor/Outer_Loop/body_to_inertial/inertial_vel_and pos_est/DT_integrator ==
  Ab : Inport
  Sum : Sum  Inputs=++|  OutDataTypeStr=single
  Sum1 : Sum  Inputs=|++  AccumDataTypeStr=single
  negate : Gain  Gain=.5*Ts  OutDataTypeStr=single
  u_delay : UnitDelay  SampleTime=-1
  u_delay1 : UnitDelay  SampleTime=-1
  Vb : Outport
  wires:
  Ab/1 -> u_delay/1, Sum/2
  u_delay/1 -> Sum/1
  Sum/1 -> negate/1
  negate/1 -> Sum1/1
  Sum1/1 -> u_delay1/1, Vb/1
  u_delay1/1 -> Sum1/2

== system Quadrotor_14_step0_code_gen/Quadrotor/Outer_Loop/body_to_inertial/inertial_vel_and pos_est/DT_integrator1 ==
  Vb : Inport
  Sum : Sum  Inputs=++|  OutDataTypeStr=single
  Sum1 : Sum  Inputs=|++  OutDataTypeStr=single
  negate : Gain  Gain=.5*Ts  OutDataTypeStr=single
  u_delay : UnitDelay  SampleTime=-1
  u_delay1 : UnitDelay  SampleTime=-1
  Xb : Outport  OutDataTypeStr=single  PortDimensions=[3]
  wires:
  u_delay1/1 -> Sum1/2
  Sum1/1 -> Xb/1, u_delay1/1
  negate/1 -> Sum1/1
  Sum/1 -> negate/1
  u_delay/1 -> Sum/1
  Vb/1 -> Sum/2, u_delay/1

== system Quadrotor_14_step0_code_gen/Quadrotor/plant_dynamics/starmac_blade_flapping_effects/starmac_body_moments/CrossProduct(AXB) ==
  A : Inport
  B : Inport  Port=2
  Fcn : Fcn  Expr=u[2]*u[6]-u[3]*u[5]
  Fcn1 : Fcn  Expr=u[3]*u[4]-u[1]*u[6]
  Fcn2 : Fcn  Expr=u[1]*u[5]-u[2]*u[4]
  Mux : Mux  Inputs=2
  Mux1 : Mux  Inputs=3
  Out : Outport
  wires:
  Mux1/1 -> Out/1
  Fcn2/1 -> Mux1/3
  Fcn1/1 -> Mux1/2
  Fcn/1 -> Mux1/1
  Mux/1 -> Fcn2/1, Fcn1/1, Fcn/1
  B/1 -> Mux/2
  A/1 -> Mux/1

== system Quadrotor_14_step0_code_gen/Quadrotor/plant_dynamics/starmac_blade_flapping_effects/starmac_body_moments/CrossProduct(AXB)1 ==
  A : Inport
  B : Inport  Port=2
  Fcn : Fcn  Expr=u[2]*u[6]-u[3]*u[5]
  Fcn1 : Fcn  Expr=u[3]*u[4]-u[1]*u[6]
  Fcn2 : Fcn  Expr=u[1]*u[5]-u[2]*u[4]
  Mux : Mux  Inputs=2
  Mux1 : Mux  Inputs=3
  Out : Outport
  wires:
  A/1 -> Mux/1
  B/1 -> Mux/2
  Mux/1 -> Fcn/1, Fcn1/1, Fcn2/1
  Fcn/1 -> Mux1/1
  Fcn1/1 -> Mux1/2
  Fcn2/1 -> Mux1/3
  Mux1/1 -> Out/1

== system Quadrotor_14_step0_code_gen/Quadrotor/plant_dynamics/starmac_blade_flapping_effects/starmac_body_moments/CrossProduct(AXB)2 ==
  A : Inport
  B : Inport  Port=2
  Fcn : Fcn  Expr=u[2]*u[6]-u[3]*u[5]
  Fcn1 : Fcn  Expr=u[3]*u[4]-u[1]*u[6]
  Fcn2 : Fcn  Expr=u[1]*u[5]-u[2]*u[4]
  Mux : Mux  Inputs=2
  Mux1 : Mux  Inputs=3
  Out : Outport
  wires:
  Mux1/1 -> Out/1
  Fcn2/1 -> Mux1/3
  Fcn1/1 -> Mux1/2
  Fcn/1 -> Mux1/1
  Mux/1 -> Fcn2/1, Fcn1/1, Fcn/1
  B/1 -> Mux/2
  A/1 -> Mux/1

== system Quadrotor_14_step0_code_gen/Quadrotor/plant_dynamics/starmac_blade_flapping_effects/starmac_body_moments/CrossProduct(AXB)3 ==
  A : Inport
  B : Inport  Port=2
  Fcn : Fcn  Expr=u[2]*u[6]-u[3]*u[5]
  Fcn1 : Fcn  Expr=u[3]*u[4]-u[1]*u[6]
  Fcn2 : Fcn  Expr=u[1]*u[5]-u[2]*u[4]
  Mux : Mux  Inputs=2
  Mux1 : Mux  Inputs=3
  Out : Outport
  wires:
  A/1 -> Mux/1
  B/1 -> Mux/2
  Mux/1 -> Fcn/1, Fcn1/1, Fcn2/1
  Fcn/1 -> Mux1/1
  Fcn1/1 -> Mux1/2
  Fcn2/1 -> Mux1/3
  Mux1/1 -> Out/1

== system Quadrotor_14_step0_code_gen/Quadrotor/plant_dynamics/starmac_blade_flapping_effects/starmac_body_moments/Motor Thrust to Torques ==
  Thrusts : Inport
  Demux : Demux
  Gain1 : Gain  Gain=K_torque
  torque 1 : Outport
  torque 2 : Outport  Port=2
  torque 3 : Outport  Port=3
  torque 4 : Outport  Port=4
  wires:
  Demux/4 -> torque 4/1
  Demux/3 -> torque 3/1
  Demux/2 -> torque 2/1
  Demux/1 -> torque 1/1
  Gain1/1 -> Demux/1
  Thrusts/1 -> Gain1/1

== matlab function Quadrotor/Outer_Loop/body_to_inertial/Ab_to_Ae ==
  data: euler input single size=[3]; Ae output single size=[3]; Ab input single size=[3]
function Ae = fcn(euler, Ab)
% This block supports the Embedded MATLAB subset.
% See the help menu for details. 
phi=euler(1);
theta=euler(2);
psi=euler(3);
c_phi=cos(phi);
c_theta=cos(theta);
c_psi=cos(psi);
s_phi=sin(phi);
s_theta=sin(theta);
s_psi=sin(psi);
R=single([c_theta*c_psi, c_theta*s_psi, -s_theta;
   s_phi*s_theta*c_psi-c_phi*s_psi, s_phi*s_theta*s_psi+c_phi*c_psi, c_theta*s_phi;
   c_phi*s_theta*c_psi+s_phi*s_psi, c_phi*s_theta*s_psi-s_phi*c_psi, c_theta*c_phi]);
%R=single(zeros(3,3));
%R(1,1)=c_theta*c_psi;
%R(1,2)=c_theta*s_psi;
%R(1,3)=-s_theta;
%R(2,1)=s_phi*s_theta*c_psi - c_phi*s_psi;
%R(2,2)=s_phi*s_theta*s_psi + c_phi*c_psi;
%R(2,3)=c_theta*s_phi;
%R(3,1)=c_phi*s_theta*c_psi + s_phi*s_psi;
%R(3,2)=c_phi*s_theta*s_psi - s_phi*c_psi;
%R(3,3)=c_theta*c_phi;
Ae= transpose(R) * Ab;
%Ae= single(Aed);

== matlab function Quadrotor/Inner_Loop/u_T_u_torque_motor_thrust/u_torque_u_T_mux ==
  data: u_torque input single size=[3]; u_torque_u_T output single size=[4]; u_T input single size=[1]
function u_torque_u_T = fcn(u_torque, u_T)
% This block supports the Embedded MATLAB subset.
% See the help menu for details. 
u_torque_u_T = [u_torque; u_T];

== matlab function Quadrotor/Outer_Loop/inertial_pos_controller/demux_fc_xyz ==
  data: fc_xyz input single size=[3]; fc_x output single size=[1]; fc_y output single size=[1]; fc_z output single size=[1]
function [fc_x,fc_y, fc_z] = fcn(fc_xyz)
% This block supports the Embedded MATLAB subset.
% See the help menu for details. 
fc_x=fc_xyz(1);
fc_y=fc_xyz(2);
fc_z=fc_xyz(3);

== matlab function Quadrotor/Outer_Loop/inertial_pos_controller/mux_euler ==
  data: ficx_ficz input single size=[1]; euler output single size=[3]; ficy_ficz input single size=[1]; psi_a input single size=[1]; psi_s input single
function euler = fcn(ficx_ficz, ficy_ficz, psi_a, psi_s)
% This block supports the Embedded MATLAB subset.
% See the help menu for details. 

A = [sin(psi_a) -cos(psi_a); cos(psi_a) sin(psi_a)];
% Get [phi, theta] 
euler_angs = (A * [ficx_ficz; ficy_ficz])';

euler=[euler_angs(1);euler_angs(2);psi_s];

== matlab function Quadrotor/Outer_Loop/rate_limiter/Embedded MATLAB Function ==
  data: Xd input single; Xr output single; Xd_prev input single; Tsamp input single; Vmax input single
function Xr = limit_rate(Xd, Xd_prev, Tsamp, Vmax)
% This block supports the Embedded MATLAB subset.
% See the help menu for details. 

delta = Xd - Xd_prev;
delta = sign(delta) .* min( abs(delta), (ones(size(delta)) * Tsamp * Vmax) );

Xr = Xd_prev + delta;

== matlab function Quadrotor/IMU/match_yaw ==
  data: u input double; y output double
function y = fcn(u)
euler_gain = 100;
if u < 0
    y = u + 360*euler_gain;
else
    y = u;
end

== matlab function Quadrotor/GPS/XY-to-lat_long/XY-to-lat_long ==
  data: XY input double size=[2]; lat output double; lon output double; lat_0 parameter double; lon_0 parameter double
function [lat,lon] = fcn(XY, lat_0, lon_0)
%Convert inertial X position and Inertial Y position to latitude and
%longitude
    R = 6371e3;          %Earth's Radius meters
    X = XY(1);           %Inertial X position meters
    Y = XY(2);           %Inertial Y position meters
    lat_0 = lat_0*pi/180;
    lon_0 = lon_0*pi/180;
    theta = atan2(Y,X);  %Radians
    d = sqrt(X^2 + Y^2); %Distance from start point (lat_0, lon_0)
    alpha = d/R;
    lat = lat_0 + alpha*cos(theta);
    if abs(theta) == pi/2
        q = cos(lat_0);
    else
        tmp = log(tan((lat/2) + (pi/4))/tan((lat_0/2) + (pi/4)));
        q = alpha*cos(theta)/tmp;
    end
    del_lon = alpha*sin(theta)/q;
    lon = mod((lon_0 + del_lon + pi),2*pi)-pi;
    lat = (180/pi)*lat; %degrees
    lon = (180/pi)*lon; %degrees
    lat = 1e7*lat; %1e-7 degrees
    lon = 1e7*lon; %1e-7 degrees

== matlab function Quadrotor/sensor_convert/convert_yaw ==
  data: u input double; y output double
function y = fcn(u)
    euler_gain = 100;
    if u > 180*euler_gain
        y = u - 360*euler_gain;
    else
        y = u;
    end

== matlab function Quadrotor/Outer_Loop/sensor_fusion/sensor_fusion ==
  data: Xe_s input double; Xe output double; Xe_f input double; Ve_s input double; Ve_f input double; Ve output double; Ts_gps parameter double; Ts parameter double
function [Xe,Ve] = fcn(Xe_s, Xe_f, Ve_s, Ve_f, Ts_gps, Ts)
%Fuse the gps measurements Xe_s and Ve_s with the
%faster inertial sensor measurements Xe_f, Ve_f
%N.B. the height is updated by a fast pressure sensor so we always
%pass through the z-component of Xe_s and Ve_s
persistent count;
persistent dXe_s_last;
persistent dVe_s_last;
persistent dXe_s_last_2;
if isempty(count)
    count = floor(Ts_gps/Ts);
    dXe_s_last = Xe_s-Xe_f;
    dXe_s_last_2 = dXe_s_last;
    dVe_s_last = Ve_s-Ve_f;
    dXe_s_last(3)=0;
    dVe_s_last(3)=0;
end
if count == floor(Ts_gps/Ts)
    count = 1; 
    temp = ((Xe_s(1:2)-Xe_f(1:2)) + dXe_s_last(1:2) + dXe_s_last_2(1:2))/3;
    dXe_s_last_2 = dXe_s_last;
    dXe_s_last(1:2) = temp;
    dVe_s_last(1:2) = Ve_s(1:2)-Ve_f(1:2);
else
    count = count + 1;
end
Xe = Xe_f + dXe_s_last;
Ve = Ve_f + dVe_s_last;
Xe(3) = Xe_s(3);
Ve(3) = Ve_s(3);

== matlab function Quadrotor/sensor_convert/lat_long-to-XY ==
  data: XY output double size=[2]; lat input double size=[1]; lon input double size=[1]
function XY  = fcn(lat,lon)
%Convert latitude and longitude to relative XY position from an initial
%latitude and longitude reading
    persistent lat_0;
    persistent lon_0;
    R = 6371e3;         %Earth's Radius meters
    lat = lat*pi/180e7; %Convert from 1e-7 degrees to radians
    lon = lon*pi/180e7; %Convert from 1e-7 degrees to radians
    if isempty(lat_0)
        lat_0 = lat;
    end
    if lat_0 == 0
        lat_0 = lat;
    end
    if isempty(lon_0)
        lon_0 = lon;
    end
    if lon_0 == 0
        lon_0 = lon;
    end
    XY = zeros(2,1);
    if (lat_0 ~= 0) && (lon_0 ~= 0)
        %Compute distance between two-points using haversine formula
        del_lat = lat - lat_0;
        del_lon = lon - lon_0;
        a = sin(del_lat/2)^2 + cos(lat)*sin(del_lon/2)^2;
        c = 2*atan2(sqrt(a),sqrt(1-a));
        d = R*c;     %Distance traveled from starting point (0,0) in meters
        yt = sin(del_lon)*cos(lat);
        xt = cos(lat_0)*sin(lat) - sin(lat_0)*cos(lat)*cos(del_lon);
        th = atan2(yt,xt);
        X = d*cos(th);
        Y = d*sin(th);
        XY(1) = X;
        XY(2) = Y;
    end
    
    lat0 = lat_0;
    lon0 = lon_0;
